simulink model "quarter_car_Active_Suspension_model"  (R2022b)
settings: Solver=ode1  StartTime=0.0  StopTime=T_f  FixedStep=0.001  MaxStep=0.1  RelTol=1e-3
values from neighbouring files (symbols this model uses):
  A = [   0       1        0          -1 ... (first row only)    [main.m]    (also in quarter_car_main.m)
  B = [  0       0 ... (first row only)    [main.m]    (also in quarter_car_main.m)
  C = [        eye(4) ... (first row only)    [main.m]    (also in quarter_car_main.m)
  D = [zeros(4,2) ... (first row only)    [main.m]    (also in quarter_car_main.m)
  K = lqr( A, B(:,2), Q, R )    [main.m]    (also in quarter_car_main.m)
  Kd = pid.Kd + 1e2    [quarter_car_main.m]
  Kd_2 = pid_2.Kd    [quarter_car_main.m]
  Ki = pid.Ki + 2*1e6    [quarter_car_main.m]
  Ki_2 = pid_2.Ki + 6*1e3    [quarter_car_main.m]
  Kp = pid.Kp + 1e5    [quarter_car_main.m]
  Kp_2 = pid_2.Kp + 1.6e2    [quarter_car_main.m]
libraries: slpidlib x2
settings Model: Creator=giacomo  LastModifiedBy=giacomo

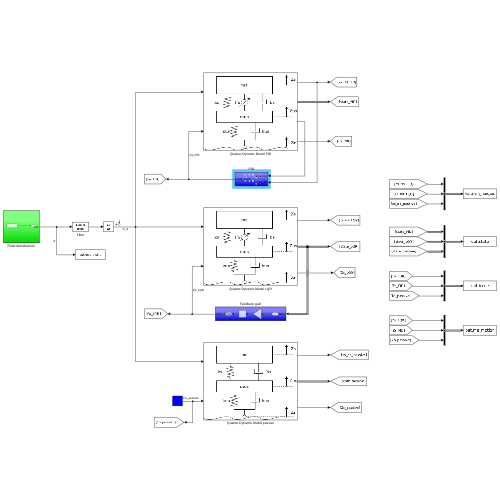
[thumbnail: Simulink's stored preview of the top-level diagram]
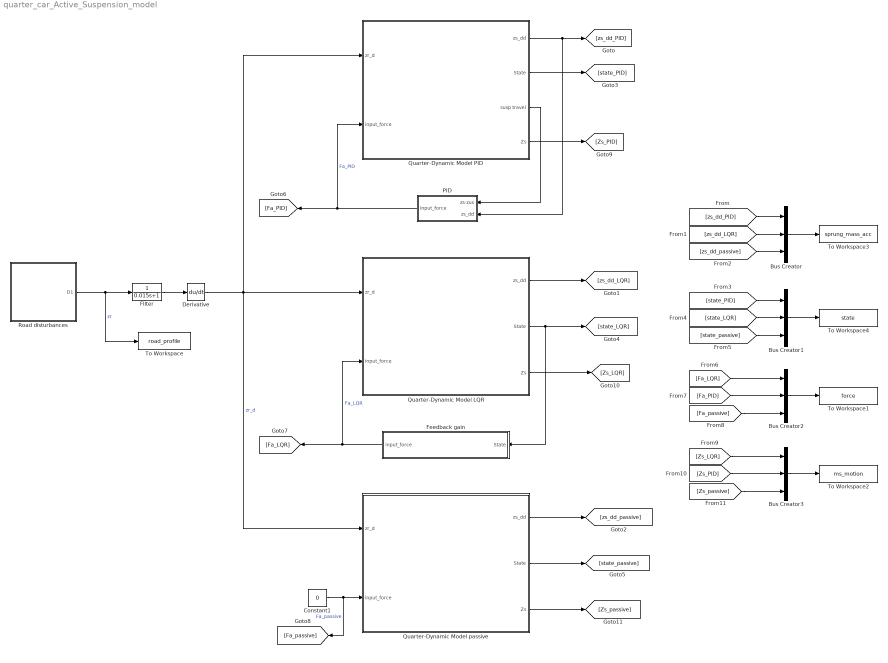
== system quarter_car_Active_Suspension_model ==
  Bus Creator{,1..3} (4 alike) : BusCreator  Inputs=3
  Constant1 : Constant  Value=0
  Derivative : Derivative
  FIlter : TransferFcn  Denominator=[0.015 1]
  Feedback gain : Subsystem
  PID : Subsystem
  Quarter-Dynamic Model LQR : Subsystem
      mask Display: image('/home/giacomo/University/Active_suspension/imgs/Active_susp.png'); % Use "Edit Image" on toolstrip to change.
  Quarter-Dynamic Model PID : Subsystem
      mask Display: image('/home/giacomo/University/Active_suspension/imgs/Active_susp.png'); % Use "Edit Image" on toolstrip to change.
  Quarter-Dynamic Model passive : Subsystem
      mask Display: image('/home/giacomo/University/Active_suspension/imgs/Passive_susp.png'); % Use "Edit Image" on toolstrip to change.
  Road disturbances : Subsystem
  To Workspace : ToWorkspace  VariableName=road_profile  SaveFormat=Timeseries  SampleTime=-1
  To Workspace1 : ToWorkspace  VariableName=force  SaveFormat=Timeseries  SampleTime=-1
  To Workspace2 : ToWorkspace  VariableName=ms_motion  SaveFormat=Timeseries  SampleTime=-1
  To Workspace3 : ToWorkspace  VariableName=sprung_mass_acc  SaveFormat=Timeseries  SampleTime=-1
  To Workspace4 : ToWorkspace  VariableName=state  SaveFormat=Timeseries  SampleTime=-1
  wires:
  Road disturbances/1(D1) -> FIlter/1, To Workspace/1  "zr"
  Constant1/1 -> [Fa_passive], Quarter-Dynamic Model passive/2(input_force)  "Fa_passive"
  Derivative/1 -> Quarter-Dynamic Model LQR/1(zr_d), Quarter-Dynamic Model PID/1(zr_d), Quarter-Dynamic Model passive/1(zr_d)  "zr_d"
  Feedback gain/1(input_force) -> [Fa_LQR], Quarter-Dynamic Model LQR/2(input_force)  "Fa_LQR"
  PID/1(input_force) -> [Fa_PID], Quarter-Dynamic Model PID/2(input_force)  "Fa_PID"
  Quarter-Dynamic Model PID/1(zs_dd) -> PID/2(zs_dd), [zs_dd_PID]
  Quarter-Dynamic Model passive/2(State) -> [state_passive]
  Quarter-Dynamic Model LQR/2(State) -> Feedback gain/1(State), [state_LQR]
  Quarter-Dynamic Model PID/2(State) -> [state_PID]
  Quarter-Dynamic Model LQR/1(zs_dd) -> [zs_dd_LQR]
  Quarter-Dynamic Model passive/1(zs_dd) -> [zs_dd_passive]
  [zs_dd_PID] -> Bus Creator/1
  [zs_dd_passive] -> Bus Creator/3
  [zs_dd_LQR] -> Bus Creator/2
  Bus Creator/1 -> To Workspace3/1
  [state_PID] -> Bus Creator1/1
  [state_LQR] -> Bus Creator1/2
  [state_passive] -> Bus Creator1/3
  Bus Creator1/1 -> To Workspace4/1
  FIlter/1 -> Derivative/1
  Quarter-Dynamic Model PID/3(susp travel) -> PID/1(zs-zus)
  [Fa_LQR] -> Bus Creator2/1
  [Fa_PID] -> Bus Creator2/2
  Bus Creator2/1 -> To Workspace1/1
  [Fa_passive] -> Bus Creator2/3
  [Zs_LQR] -> Bus Creator3/1
  [Zs_PID] -> Bus Creator3/2
  Bus Creator3/1 -> To Workspace2/1
  [Zs_passive] -> Bus Creator3/3
  Quarter-Dynamic Model PID/4(Zs) -> [Zs_PID]
  Quarter-Dynamic Model LQR/3(Zs) -> [Zs_LQR]
  Quarter-Dynamic Model passive/3(Zs) -> [Zs_passive]

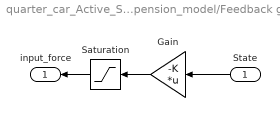
== system quarter_car_Active_Suspension_model/Feedback gain ==
  State : Inport
  Gain : Gain  Gain=-K  Multiplication=Matrix(K*u)
  Saturation : Saturate  UpperLimit=46730  LowerLimit=-46730
  input_force : Outport
  wires:
  State/1 -> Gain/1
  Gain/1 -> Saturation/1
  Saturation/1 -> input_force/1

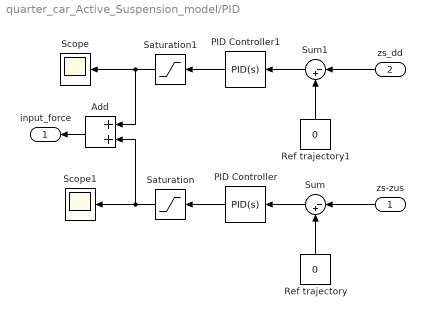
== system quarter_car_Active_Suspension_model/PID ==
  zs-zus : Inport
  zs_dd : Inport  Port=2
  Add : Sum
  PID Controller : slpidlib/PID Controller  Controller=PID  Form=Parallel  TimeDomain=Continuous-time  UseExternalTs=off  SampleTime=-1  IntegratorMethod=Forward Euler  FilterMethod=Forward Euler  ControllerParametersSource=internal  P=Kp  I=Ki  UseKiTs=off  D=Kd  N=1000  UseFilter=on  TunerSelectOption=Transfer Function Based (PID Tuner App)  InitialConditionSource=internal  InitialConditionForIntegrator=0  InitialConditionForFilter=0  DifferentiatorICPrevScaledInput=0  ExternalReset=none  TrackingMode=off  Kt=1  LimitOutput=off  SatLimitsSource=internal  UpperSaturationLimit=inf  LowerSaturationLimit=-inf  LinearizeAsGain=on  AntiWindupMode=none  Kb=1  LimitIntegrator=off  UpperIntegratorSaturationLimit=inf  LowerIntegratorSaturationLimit=-inf  POutMin=[]  POutMax=[]  IOutMin=[]  IOutMax=[]  DOutMin=[]  DOutMax=[]  NOutMin=[]  NOutMax=[]  SumOutMin=[]  SumOutMax=[]  SaturationOutMin=[]  SaturationOutMax=[]  PParamMin=[]  PParamMax=[]  IParamMin=[]  IParamMax=[]  DParamMin=[]  DParamMax=[]  NParamMin=[]  NParamMax=[]  KbParamMin=[]  KbParamMax=[]  KtParamMin=[]  KtParamMax=[]  KbOutMin=[]  KbOutMax=[]  KtOutMin=[]  KtOutMax=[]  IntegratorOutMin=[]  IntegratorOutMax=[]  FilterOutMin=[]  FilterOutMax=[]  SumI1OutMin=[]  SumI1OutMax=[]  SumI2OutMin=[]  SumI2OutMax=[]  SumI3OutMin=[]  SumI3OutMax=[]  SumI4OutMin=[]  SumI4OutMax=[]  SumDOutMin=[]  SumDOutMax=[]  DifferentiatorOutMin=[]  DifferentiatorOutMax=[]  FilterDiffOutCoefMin=[]  FilterDiffOutCoefMax=[]  ReciprocalOutMin=[]  ReciprocalOutMax=[]  SumDenOutMin=[]  SumDenOutMax=[]  SumNumOutMin=[]  SumNumOutMax=[]  DivideOutMin=[]  DivideOutMax=[]  UdiffTsProdOutMin=[]  UdiffTsProdOutMax=[]  NTsProdOutMin=[]  NTsProdOutMax=[]  UintegralTsProdOutMin=[]  UintegralTsProdOutMax=[]  UngainTsProdOutMin=[]  UngainTsProdOutMax=[]  ClampingZeroOutDataTypeStr=Inherit: Inherit via back propagation  ClampingZeroOutMin=[]  ClampingZeroOutMax=[]  FilterDenConstantOutDataTypeStr=Inherit: Inherit via back propagation  FilterDenConstantOutMin=[]  FilterDenConstantOutMax=[]  PCopyOutDataTypeStr=Inherit: Inherit via back propagation  PCopyOutMin=[]  PCopyOutMax=[]  NCopyOutDataTypeStr=Inherit: Inherit via back propagation  NCopyOutMin=[]  NCopyOutMax=[]  IntegratorContinuousStateAttributes=''  IntegratorStateMustResolveToSignalObject=off  IntegratorRTWStateStorageClass=Auto  FilterContinuousStateAttributes=''  FilterStateMustResolveToSignalObject=off  FilterRTWStateStorageClass=Auto  ParallelPVariant=InternalParameters  IdealPVariant=Disabled  IVariant=InternalParameters  DVariant=InternalParameters  IntegratorVariant=Continuous  SatVariant=Disabled  AWVariant=Passthrough  PCopyVariant=Disabled  TRVariant=Disabled  FdbkBlocksVariant=Forward  IdealPFdbkVariant=Disabled  SatFdbkVariant=Disabled  DerivativeFilterVariant=ContFilter  NVariant=InternalParameters  NCopyVariant=Disabled  FilterICVariant=InternalICsFilter  IntegratorICVariant=InternalICs  ExternalResetVariant=Disabled  TRSumVariant=Passthrough  SumFdbkVariant=Disabled  SumVariant=Sum_PID  TsampFilterVariant=InternalTs  TsampNgainVariant=Passthrough  TsampIntegralVariant=Passthrough  ExternalSaturationOutDataTypeStr=Inherit: Same as second input
  PID Controller1 : slpidlib/PID Controller  Controller=PID  Form=Parallel  TimeDomain=Continuous-time  UseExternalTs=off  SampleTime=-1  IntegratorMethod=Forward Euler  FilterMethod=Forward Euler  ControllerParametersSource=internal  P=Kp_2  I=Ki_2  UseKiTs=off  D=Kd_2  N=1000  UseFilter=on  TunerSelectOption=Transfer Function Based (PID Tuner App)  InitialConditionSource=internal  InitialConditionForIntegrator=0  InitialConditionForFilter=0  DifferentiatorICPrevScaledInput=0  ExternalReset=none  TrackingMode=off  Kt=1  LimitOutput=off  SatLimitsSource=internal  UpperSaturationLimit=inf  LowerSaturationLimit=-inf  LinearizeAsGain=on  AntiWindupMode=none  Kb=1  LimitIntegrator=off  UpperIntegratorSaturationLimit=inf  LowerIntegratorSaturationLimit=-inf  POutMin=[]  POutMax=[]  IOutMin=[]  IOutMax=[]  DOutMin=[]  DOutMax=[]  NOutMin=[]  NOutMax=[]  SumOutMin=[]  SumOutMax=[]  SaturationOutMin=[]  SaturationOutMax=[]  PParamMin=[]  PParamMax=[]  IParamMin=[]  IParamMax=[]  DParamMin=[]  DParamMax=[]  NParamMin=[]  NParamMax=[]  KbParamMin=[]  KbParamMax=[]  KtParamMin=[]  KtParamMax=[]  KbOutMin=[]  KbOutMax=[]  KtOutMin=[]  KtOutMax=[]  IntegratorOutMin=[]  IntegratorOutMax=[]  FilterOutMin=[]  FilterOutMax=[]  SumI1OutMin=[]  SumI1OutMax=[]  SumI2OutMin=[]  SumI2OutMax=[]  SumI3OutMin=[]  SumI3OutMax=[]  SumI4OutMin=[]  SumI4OutMax=[]  SumDOutMin=[]  SumDOutMax=[]  DifferentiatorOutMin=[]  DifferentiatorOutMax=[]  FilterDiffOutCoefMin=[]  FilterDiffOutCoefMax=[]  ReciprocalOutMin=[]  ReciprocalOutMax=[]  SumDenOutMin=[]  SumDenOutMax=[]  SumNumOutMin=[]  SumNumOutMax=[]  DivideOutMin=[]  DivideOutMax=[]  UdiffTsProdOutMin=[]  UdiffTsProdOutMax=[]  NTsProdOutMin=[]  NTsProdOutMax=[]  UintegralTsProdOutMin=[]  UintegralTsProdOutMax=[]  UngainTsProdOutMin=[]  UngainTsProdOutMax=[]  ClampingZeroOutDataTypeStr=Inherit: Inherit via back propagation  ClampingZeroOutMin=[]  ClampingZeroOutMax=[]  FilterDenConstantOutDataTypeStr=Inherit: Inherit via back propagation  FilterDenConstantOutMin=[]  FilterDenConstantOutMax=[]  PCopyOutDataTypeStr=Inherit: Inherit via back propagation  PCopyOutMin=[]  PCopyOutMax=[]  NCopyOutDataTypeStr=Inherit: Inherit via back propagation  NCopyOutMin=[]  NCopyOutMax=[]  IntegratorContinuousStateAttributes=''  IntegratorStateMustResolveToSignalObject=off  IntegratorRTWStateStorageClass=Auto  FilterContinuousStateAttributes=''  FilterStateMustResolveToSignalObject=off  FilterRTWStateStorageClass=Auto  ParallelPVariant=InternalParameters  IdealPVariant=Disabled  IVariant=InternalParameters  DVariant=InternalParameters  IntegratorVariant=Continuous  SatVariant=Disabled  AWVariant=Passthrough  PCopyVariant=Disabled  TRVariant=Disabled  FdbkBlocksVariant=Forward  IdealPFdbkVariant=Disabled  SatFdbkVariant=Disabled  DerivativeFilterVariant=ContFilter  NVariant=InternalParameters  NCopyVariant=Disabled  FilterICVariant=InternalICsFilter  IntegratorICVariant=InternalICs  ExternalResetVariant=Disabled  TRSumVariant=Passthrough  SumFdbkVariant=Disabled  SumVariant=Sum_PID  TsampFilterVariant=InternalTs  TsampNgainVariant=Passthrough  TsampIntegralVariant=Passthrough  ExternalSaturationOutDataTypeStr=Inherit: Same as second input
  Ref trajectory : Constant  Value=0
  Ref trajectory1 : Constant  Value=0
  Saturation : Saturate  UpperLimit=46730  LowerLimit=-46730
  Saturation1 : Saturate  UpperLimit=46730  LowerLimit=-46730
  Scope : Scope
  Scope1 : Scope
  Sum : Sum  Inputs=|-+
  Sum1 : Sum  Inputs=|-+
  input_force : Outport
  wires:
  Sum/1 -> PID Controller/1
  zs-zus/1 -> Sum/1
  PID Controller/1 -> Saturation/1
  Ref trajectory/1 -> Sum/2
  Ref trajectory1/1 -> Sum1/2
  PID Controller1/1 -> Saturation1/1
  Sum1/1 -> PID Controller1/1
  Add/1 -> input_force/1
  Saturation1/1 -> Scope/1, Add/1
  Saturation/1 -> Scope1/1, Add/2
  zs_dd/1 -> Sum1/1

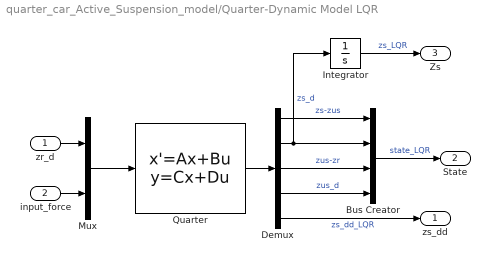
== system quarter_car_Active_Suspension_model/Quarter-Dynamic Model LQR ==
  zr_d : Inport
  input_force : Inport  Port=2
  Bus Creator : BusCreator  Inputs=4
  Demux : Demux  Outputs=5
  Integrator : Integrator
  Mux : Mux  Inputs=2
  Quarter : StateSpace  A=A  B=B  C=C  D=D  InitialCondition=0
  zs_dd : Outport
  State : Outport  Port=2
  Zs : Outport  Port=3
  wires:
  Mux/1 -> Quarter/1
  zr_d/1 -> Mux/1
  input_force/1 -> Mux/2
  Quarter/1 -> Demux/1
  Demux/1 -> Bus Creator/1  "zs-zus"
  Demux/2 -> Integrator/1, Bus Creator/2  "zs_d"
  Demux/3 -> Bus Creator/3  "zus-zr"
  Demux/4 -> Bus Creator/4  "zus_d"
  Bus Creator/1 -> State/1  "state_LQR"
  Demux/5 -> zs_dd/1  "zs_dd_LQR"
  Integrator/1 -> Zs/1  "zs_LQR"

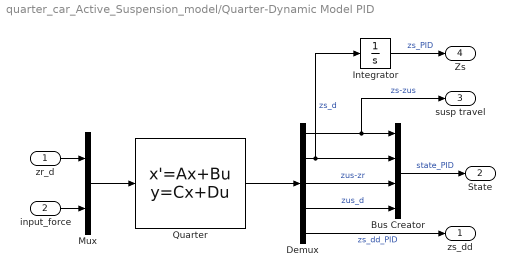
== system quarter_car_Active_Suspension_model/Quarter-Dynamic Model PID ==
  zr_d : Inport
  input_force : Inport  Port=2
  Bus Creator : BusCreator  Inputs=4
  Demux : Demux  Outputs=5
  Integrator : Integrator
  Mux : Mux  Inputs=2
  Quarter : StateSpace  A=A  B=B  C=C  D=D  InitialCondition=0
  zs_dd : Outport
  State : Outport  Port=2
  susp travel : Outport  Port=3
  Zs : Outport  Port=4
  wires:
  Mux/1 -> Quarter/1
  zr_d/1 -> Mux/1
  input_force/1 -> Mux/2
  Demux/3 -> Bus Creator/3  "zus-zr"
  Demux/1 -> Bus Creator/1, susp travel/1  "zs-zus"
  Demux/2 -> Bus Creator/2, Integrator/1  "zs_d"
  Bus Creator/1 -> State/1  "state_PID"
  Quarter/1 -> Demux/1
  Demux/4 -> Bus Creator/4  "zus_d"
  Demux/5 -> zs_dd/1  "zs_dd_PID"
  Integrator/1 -> Zs/1  "zs_PID"

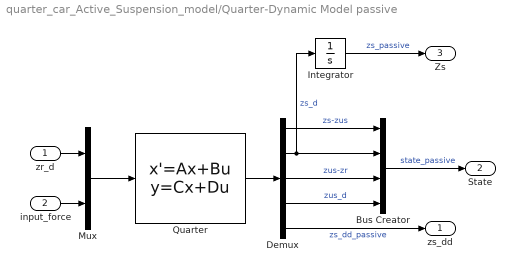
== system quarter_car_Active_Suspension_model/Quarter-Dynamic Model passive ==
  zr_d : Inport
  input_force : Inport  Port=2
  Bus Creator : BusCreator  Inputs=4
  Demux : Demux  Outputs=5
  Integrator : Integrator
  Mux : Mux  Inputs=2
  Quarter : StateSpace  A=A  B=B  C=C  D=D  InitialCondition=0
  zs_dd : Outport
  State : Outport  Port=2
  Zs : Outport  Port=3
  wires:
  Mux/1 -> Quarter/1
  zr_d/1 -> Mux/1
  input_force/1 -> Mux/2
  Demux/3 -> Bus Creator/3  "zus-zr"
  Demux/2 -> Bus Creator/2, Integrator/1  "zs_d"
  Quarter/1 -> Demux/1
  Bus Creator/1 -> State/1  "state_passive"
  Demux/4 -> Bus Creator/4  "zus_d"
  Demux/1 -> Bus Creator/1  "zs-zus"
  Demux/5 -> zs_dd/1  "zs_dd_passive"
  Integrator/1 -> Zs/1  "zs_passive"

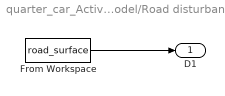
== system quarter_car_Active_Suspension_model/Road disturbances ==
  From Workspace : FromWorkspace  VariableName=road_surface
  D1 : Outport
  wires:
  From Workspace/1 -> D1/1
